simulink library "DSCdq_Library"  (R2018a)
settings: Solver=VariableStepAuto  StartTime=0.0  StopTime=10.0  RelTol=1e-3
values from neighbouring files (symbols this model uses):
  Fcutout = 1000    [Application_Script.m]
  Fmin = 40    [Application_Script.m]
  Fn = 60    [Application_Script.m]    (also in ShortPulse_Script.m)
  Fsw = 6000    [Application_Script.m]
  Kp = 4    [Application_Script.m]
  Ti = L/R    (= 0.0530516476973)    [Application_Script.m]
  Ts = Ts_control / 60    (= 9.25925925926e-07)    [Application_Script.m]    (also in ShortPulse_Script.m)
  Ts_control = 1/(300*Fn)    (= 5.55555555556e-05)    [Application_Script.m]    (also in ShortPulse_Script.m)
  X = 0.5    [Application_Script.m]
  zeta = 2^-0.5    (= 0.707106781187)    [Application_Script.m]    (also in ShortPulse_Script.m)
undefined symbols (not defined in the file or in its folder): DiscIntNeverNeededParam, ESS, fn, Iap, PCC, Sn, tctrl, Uanp
libraries: $bdroot x54, powerlib_meascontrol x33, powerlib x3, cstblocks x2, simulink x2, peTransforms x2
(part 1 of 2)
settings Model: Creator=daniemot  LastModifiedBy=daniemot

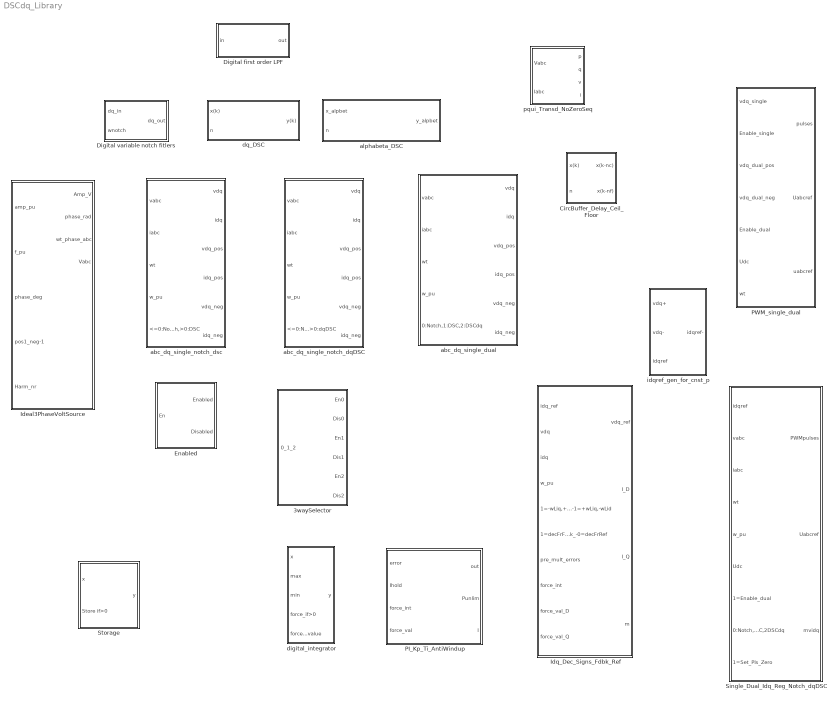
== system DSCdq_Library ==
  3waySelector : Subsystem  SystemSampleTime=Ts  mask(3 way selector){}
      mask Display: fprintf('Selector');
  CircBuffer_Delay_Ceil_Floor : Subsystem  TreatAsAtomicUnit=on  SystemSampleTime=Ts  mask(Circular buffer with two variable delays (ceiling and floor)){Ts=Ts, nmax=200}
      mask prompts: Ts "Sampling time [s]"; nmax "Circular buffer length"
      mask help:
      | Circular Buffer
      | By: Mota
      | Revision history:	2021-07-16: first release
      |
      | Interface
      | Inputs
      | 	x : must be a vector pf two values
      | 	n : delay in samples (float, ideal delay is time was continuous)
      | 	nmax : max size of circular buffer, ONLY used in FIRST CYCLE
      |
      | Output
      | 	yc = x(k - ceil(n))
      | 	yf = x(k - floor(n))
  Digital first order LPF : Subsystem  mask(Digital first-order low-pass filter){Ts=tctrl, fcutout=fn/2^0.5}
      mask prompts: Ts "Sample times [s]"; fcutout "Cutout frequency [Hz]"
      mask help:
      | Continuous time transfer function:  1/(1 + s T)
      | 	where T [s] = 1 / (2 pi fcutout [Hz]).
      |
      | Actual digital transfer function:   alpha / (1 + ( alpha -1) z^{-1} )
      | 	with eq. of diffs.: y = alpha x + (1 - alpha) y z^{-1}
      | 	where alpha = Ts / ( 1/(2 pi fcutout) + Ts)
      mask Display: fprintf('1/(1+sT)');
  Digital variable notch fitlers : Subsystem  mask{Ts=Ts, zeta=0.707}
      mask prompts: Ts "Sampling time [s]"; zeta "Damping factor zeta for notches"
  Enabled : Subsystem  SystemSampleTime=Ts  mask(Enabled block){}
      mask help:
      | if En > 0
      |     Enabled = 1;
      |     Disabled = 0;
      | else
      |     Enabled = 0;
      |     Disabled = 1;
      | end
      mask Display: fprintf('Enable');
  Ideal3PhaseVoltSource : Subsystem  mask(Three-phase ideal voltage source){BaseAmp=1, fn=50}
      mask prompts: BaseAmp "Base phase-to-neutral amplitude [V]"; fn "Base frequency [Hz]"
      mask help:
      | Three-phase balanced ideal voltage source with neutral point not connected.
      |
      | The voltage source can be connected in series with others.
      |
      | va [V] = amp_pu*BaseAmp*sin(2*pi*(f_pu/s)*Harm_nr + Harm_nr*phase_deg*pi/180)
      | vb [V] = ... + Harm_nr*Ph_b_sign*2*pi/3)
      | vc [V] = ... + Harm_nr*Ph_c_sign*2*pi/3)
      |
      | If Pos1_Neg-1 = 1
      | 	Ph_b_sign = -1
      | 	Ph_c_sign = +1
      |
      | If Pos1_Neg-1 = -1
      | 	Ph_b_sign = +1
      | 	Ph_c_sign = -1
  Idq_Dec_Signs_Fdbk_Ref : Subsystem  mask(Idq Controller - PI regulator with anti-windup){Ts=Ts_control, fn=50, Kp=0.4, Ti=0.13, L=0.3, PI_max=1.5, PI_min=-1.5, TrafoPhaseComp=0}
      mask prompts: Ts "Sampling time [s]"; fn "Rated frequency: fn [Hz]"; Kp "Proportional gain: Kp [pu]"; Ti "Integral time: Ti [s]"; L "DQ decoupl. inductance: L [pu]"; PI_max "Maximum output [pu]"; PI_min "Minimum output [pu]"; TrafoPhaseComp "Transformer phase compensation [rad]"
      mask help:
      | Idq Controller
      | Discrete PI regulator with forward Euler approximation for the integrator.
      | Transfer function: 	Kp (1 + sTi) / (sTi)
      | The anti-windup freezes the integrator if the unlimited output of the PI goes beyond the limits.
      |
      | Phase compensation for transformer winding: PhaseTrafoComp
  PI_Kp_Ti_AntiWindup : Subsystem  TreatAsAtomicUnit=on  SystemSampleTime=Ts  mask(PI regulator with anti-windup){Ts=0.001, Kp=10, Ti=1, PI_max=1, PI_min=-1}
      mask prompts: Ts "Sampling time [s]"; Kp "Proportional gain: Kp [pu]"; Ti "Integral time: Ti [s]"; PI_max "Maximum output [pu]"; PI_min "Minimum output [pu]"
      mask help:
      | Discrete PI regulator with forward Euler approximation for the integrator.
      |
      | Transfer function:
      | 	Kp (1 + sTi) / (sTi)
      |
      | The anti-windup freezes the integrator if the unlimited output of the PI goes beyond the limits.
      mask Display: fprintf('Kp(1+1/(sTi))');
  PWM_single_dual : Subsystem  mask(Scaling of vdq ref and PWM gate generation){fsw=50, Ts=1/200000, Uabp=1000, PWM_Ini_Phase=90}
      mask prompts: fsw "Switching frequency [Hz]"; Ts "Sampling time [s]"; Uabp "Rated peak line voltage [V]"; PWM_Ini_Phase "PWM carrier initial phase [degrees]"
      mask help:
      | Scales vdq_ref by: U_line_peak / Udc
      |
      | Add third harmonic to uabc_ref for overmodulation
  Single_Dual_Idq_Reg_Notch_dqDSC : Subsystem  mask(Notch based dual dq current regulator){Ts=Ts_control, fgrid=Fn, fmin=Fmin, zetanotch=zeta, fcutout=Fcutout, PI_Kp=Kp, PI_Ti=Ti, PI_X=X, PI_max=1.5, PI_min=-1.5, PWM_Ts=Ts, PWM_fsw=Fsw, PWM_Uabp=3^0.5, PWM_Ini=90}
      mask prompts: Ts "Sampling time controller [s]"; fgrid "Grid frequency [Hz]"; fmin "Min. acceptable grid freq. [Hz]"; zetanotch "Damping notch filters"; fcutout "Cutout freq. low pass for noise [Hz]"; PI_Kp "Proportional gain Kp [pu/pu]"; PI_Ti "Integrator time Ti [s]"; PI_X "Decoupling reactance X [pu]"; PI_max "PI max [pu]"; PI_min "PI min [pu]"; PWM_Ts "Sampling time PWM [s]"; PWM_fsw "Switching frequency [Hz]"; PWM_Uabp "Rated peak line voltage [V]"; PWM_Ini "Initial phase of carrier [degrees]"
      mask help: To be used with "abc -> dq" and "acb -> dq" transformations. When va = V sin (wt), vb = V sin (wt-120), vc = V sin (wt+120), -> vd = V vq=0.
      mask DialogControl Container2 Prompt: Transducers
      mask DialogControl Container7 Prompt: PI regulator
      mask DialogControl Container5 Prompt: PWM
  Storage : Subsystem  SystemSampleTime=Ts  mask(Storage block){}
      mask help:
      | if Store ==1
      |     Output = Input;
      | else
      |     Output = old ouptut;
      | end
      mask Display: fprintf('Store');
  abc_dq_single_dual : Subsystem  mask(abc->dq with Matlab){Ts=0.001, fn=50, fmin=40, zeta=0.707}
      mask prompts: Ts "Sampling time [s]"; fn "Grid frequency [Hz]"; fmin "Min. acceptable grid freq. [Hz]"; zeta "Zeta for notch filters"
      mask help:
      | To be done
      |
      | Max buffer size for DSC 500 samples
  abc_dq_single_notch_dqDSC : Subsystem  mask(abc->dq with Matlab){Ts=0.001, fn=50, fmin=40, zeta=0.707}
      mask prompts: Ts "Sampling time [s]"; fn "Grid frequency [Hz]"; fmin "Min. acceptable grid freq. [Hz]"; zeta "Zeta for notch filters"
      mask help:
      | To be done
      |
      | Max buffer size for DSC 500 samples
  abc_dq_single_notch_dsc : Subsystem  mask(abc->dq with Matlab){Ts=0.001, fn=50, fmin=40, zeta=0.707}
      mask prompts: Ts "Sampling time [s]"; fn "Rated grid frequency [Hz]"; fmin "Min. acceptable grid freq. [Hz]"; zeta "Zeta for notch filters"
      mask help:
      | To be done
      |
      | Max buffer size for DSC 500 samples
  alphabeta_DSC : Subsystem  mask{Ts=Ts, nmax=200}
      mask prompts: Ts "Sample times [s]"; nmax "Maximum delay nmax:"
      mask Display: fprintf('y(k)=0.5(x(k)+jx(k-n))');
  digital_integrator : Subsystem  SystemSampleTime=Ts  mask(Digital integrator){Ts=tctrl}
      mask prompts: Ts "Sample times [s]"
      mask help:
      | Forward Euler method: as in matlab help
      | 	y(n) = y(n-1) + Ts(n-1)*x(n-1)
      | uset it to avoid algebraic loops
      |
      | All inputs are stored in states, so there is no direct feedthrough. GAMBIARRA for avoiding algebraic loops, see https://www.mathworks.com/help/simulink/ug/integration-considerations-for-matlab-function-blocks.html
      |
      | Inputs
      |    x: input to the integrator
      |    max: max value for integrator
      |    min: min value for integrator
      |    force: if>=1 sets integrator to forceval
      |    forceval: see line above (max and min are respected
      |    Ts: sampling time
      | Output
      |    y: output of the integrator
      mask Display: fprintf('1/s');
  dq_DSC : Subsystem  mask{Ts=Ts, nmax=200}
      mask prompts: Ts "Sample times [s]"; nmax "Maximum delay nmax:"
      mask Display: fprintf('y(k)=0.5(x(k)+x(k-n))');
  idqref_gen_for_cnst_p : Subsystem  mask(idq reference gen for neg. seq. controller){Ts_control=Ts_control}
      mask prompts: Ts_control "Sampling time [s]"
      mask help:
      | Calculation of the negative sequence references for removing active power second harmonic oscillations.
      | Reactive power is allowed to oscillated with second harmonic.
      |
      | To be used with "abc -> dq" and "acb -> dq" transformations. When va = V sin (wt), vb = V sin (wt-120), vc = V sin (wt+120), -> vd = V vq=0.
      |
      | In "expanded" matrix form
      | | idn | = - | -vdp  +vqp |^{-1} * | -vdn  +vqn | * | idp |
      | | iqn | =   | +vqp  +vdp |        | -vdn  +vqn |   | idq |
      | In matrix form
      | idqn  = - vdqp^{-1} * vdqn * idqp
      |
      | Not tested for "abc (-omega) -> dq" (which I think is the formulation of Chaudhary 2012.
      | Derived independently from, but later noticed that it was proposed by Chaudhary in 2012 at "Negative Sequence Current Control in Wind Power Plants With VSC-HVDC Connection", check eq. (11).
  pqui_Transd_NoZeroSeq : Subsystem  mask(u i p q transducer - No zero sequence){Sn=Sn, Uanp=Uanp, Iap=Iap}
      mask prompts: Sn "Rated three-phase apparent power [VA]"; Uanp "Rated peak phase-to-groud voltage [V]"; Iap "Rated peak line current [A]"
      mask help:
      | Loosely based on Akagi 1984, but with Clarke Transformation for both the current and voltage
      | 	v  = (valpha^2 + vbeta^2)^0.5 / V_phase_peak
      | 	i   = (ialpha^2 + ibeta^2)^0.5 / I_line_peak
      | 	p  = 3/2 * (valpha ialpha +vbeta ibeta) / Sn
      | 	q  = 3/2 * (-valpha ibeta +vbeta ialpha) / Sn

== system DSCdq_Library/3waySelector ==
  0_1_2 : Inport
  MATLAB Function : MATLAB Function  SystemSampleTime=Ts
      settings: RTWSystemCode=Inline
  En0 : Outport
  Dis0 : Outport  Port=2
  En1 : Outport  Port=3
  Dis1 : Outport  Port=4
  En2 : Outport  Port=5
  Dis2 : Outport  Port=6
  wires:
  0_1_2/1 -> MATLAB Function/1(In)
  MATLAB Function/1(En0) -> En0/1
  MATLAB Function/2(Dis0) -> Dis0/1
  MATLAB Function/3(En1) -> En1/1
  MATLAB Function/4(Dis1) -> Dis1/1
  MATLAB Function/5(En2) -> En2/1
  MATLAB Function/6(Dis2) -> Dis2/1

== system DSCdq_Library/CircBuffer_Delay_Ceil_Floor ==
  x(k) : Inport
  n : Inport  Port=2
  Constant1 : Constant  Value=nmax
  MATLAB Function : MATLAB Function  TreatAsAtomicUnit=on  SystemSampleTime=Ts
  x(k-nc) : Outport
  x(k-nf) : Outport  Port=2
  wires:
  n/1 -> MATLAB Function/2(n)  "n"
  MATLAB Function/2(yf) -> x(k-nf)/1  "x(k-nf)"
  x(k)/1 -> MATLAB Function/1(x)  "x(k)"
  MATLAB Function/1(yc) -> x(k-nc)/1  "x(k-nc)"
  Constant1/1 -> MATLAB Function/3(nmax)

== system DSCdq_Library/Digital first order LPF ==
  note: Transfer function: alpha / ( 1 + ( alpha -1 ) z^{-1} )
  note: alpha = Ts / ( 1/(2 pi fcutout) + Ts )
  note: y = alpha x + ( 1 - alpha) y z^{-1}
  in : Inport
  Add7 : Sum  Commented=on  Inputs=+-
  Discrete Filter : DiscreteFilter  Numerator=[Ts/(1/(2*pi*fcutout)+Ts)]  Denominator=[1 Ts/(1/(2*pi*fcutout)+Ts)-1]  SampleTime=Ts
  Discrete-Time Integrator : DiscreteIntegrator  Commented=on  IntegratorMethod=Integration: Trapezoidal  SampleTime=Ts  ICPrevOutput=DiscIntNeverNeededParam  ICPrevScaledInput=DiscIntNeverNeededParam
  Gain6 : Gain  Commented=on  Gain=2*pi*fcutout
  Rate Transition3 : RateTransition  OutPortSampleTime=Ts
  out : Outport
  wires:
  Add7/1 -> Gain6/1
  Discrete-Time Integrator/1 -> Add7/2
  in/1 -> Rate Transition3/1
  Gain6/1 -> Discrete-Time Integrator/1
  Rate Transition3/1 -> Add7/1, Discrete Filter/1
  Discrete Filter/1 -> out/1

== system DSCdq_Library/Digital variable notch fitlers ==
  dq_in : Inport
  wnotch : Inport  Port=2
  Constant : Constant  Value=0
  Constant1 : Constant  Value=zeta
  Constant2 : Constant  Value=0
  Constant3 : Constant  Value=zeta
  Demux : Demux  Outputs=2
  Discrete Varying Notch : cstblocks/Linear Parameter Varying/Discrete Varying Notch  w0=0  Ts=Ts
      settings: SourceProductName=Control System Toolbox  SourceProductBaseCode=CT
  Discrete Varying Notch1 : cstblocks/Linear Parameter Varying/Discrete Varying Notch  w0=0  Ts=Ts
      settings: SourceProductName=Control System Toolbox  SourceProductBaseCode=CT
  Mux : Mux  Inputs=2
  dq_out : Outport
  wires:
  Constant/1 -> Discrete Varying Notch/3
  Constant1/1 -> Discrete Varying Notch/4
  Demux/2 -> Discrete Varying Notch1/1
  dq_in/1 -> Demux/1
  Constant2/1 -> Discrete Varying Notch1/3
  wnotch/1 -> Discrete Varying Notch1/2, Discrete Varying Notch/2
  Constant3/1 -> Discrete Varying Notch1/4
  Demux/1 -> Discrete Varying Notch/1
  Discrete Varying Notch/1 -> Mux/1
  Mux/1 -> dq_out/1
  Discrete Varying Notch1/1 -> Mux/2

== system DSCdq_Library/Enabled ==
  En : Inport
  MATLAB Function : MATLAB Function  SystemSampleTime=Ts
      settings: RTWSystemCode=Inline
  Enabled : Outport
  Disabled : Outport  Port=2
  wires:
  En/1 -> MATLAB Function/1(En)
  MATLAB Function/1(Enabled) -> Enabled/1
  MATLAB Function/2(Disabled) -> Disabled/1

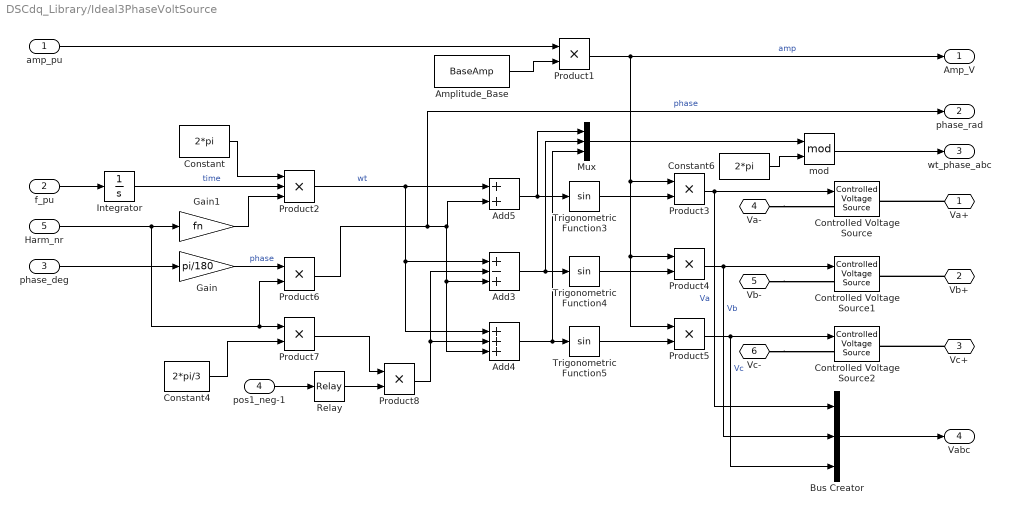
== system DSCdq_Library/Ideal3PhaseVoltSource ==
  amp_pu : Inport
  f_pu : Inport  Port=2
  phase_deg : Inport  Port=3
  pos1_neg-1 : Inport  Port=4
  Harm_nr : Inport  Port=5
  Add3 : Sum  Inputs=+-+
  Add4 : Sum  Inputs=+++
  Add5 : Sum
  Amplitude_Base : Constant  Value=BaseAmp
  Bus Creator : BusCreator  Inputs=3
  Constant : Constant  Value=2*pi
  Constant4 : Constant  Value=2*pi/3
  Constant6 : Constant  Value=2*pi
  Controlled Voltage Source : powerlib/Electrical Sources/Controlled Voltage Source  Initialize=off  Source_Type=AC  Amplitude=ESS.LSC.Ub*(2/3)^0.5  Phase=0  Frequency=PCC.fn  Measurements=None
  Controlled Voltage Source1 : powerlib/Electrical Sources/Controlled Voltage Source  Initialize=off  Source_Type=AC  Amplitude=ESS.LSC.Ub*(2/3)^0.5  Phase=-120  Frequency=PCC.fn  Measurements=None
  Controlled Voltage Source2 : powerlib/Electrical Sources/Controlled Voltage Source  Initialize=off  Source_Type=AC  Amplitude=ESS.LSC.Ub*(2/3)^0.5  Phase=120  Frequency=PCC.fn  Measurements=None
  Gain : Gain  Gain=pi/180
  Gain1 : Gain  Gain=fn
  Integrator : Integrator
  Mux : Mux  Inputs=3
  Product{1,3..8} (7 alike) : Product
  Product2 : Product  Inputs=3
  Relay : Relay  OnSwitchValue=0  OffSwitchValue=-0.1  OffOutputValue=-1
  Trigonometric Function3 : Trigonometry
  Trigonometric Function4 : Trigonometry
  Trigonometric Function5 : Trigonometry
  mod : Math  Operator=mod  SaturateOnIntegerOverflow=on
  Va+ : PMIOPort  Side=Right
  Vb+ : PMIOPort  Port=2  Side=Right
  Vc+ : PMIOPort  Port=3  Side=Right
  Va- : PMIOPort  Port=4  Side=Right
  Vb- : PMIOPort  Port=5  Side=Right
  Vc- : PMIOPort  Port=6  Side=Right
  Amp_V : Outport
  phase_rad : Outport  Port=2
  wt_phase_abc : Outport  Port=3
  Vabc : Outport  Port=4
  wires:
  Add4/1 -> Mux/3, Trigonometric Function5/1
  Product6/1 -> phase_rad/1, Add4/3, Add3/3, Add5/2  "phase"
  Add3/1 -> Mux/2, Trigonometric Function4/1
  pos1_neg-1/1 -> Relay/1
  Product3/1 -> Bus Creator/1, Controlled Voltage Source/1  "Va"
  amp_pu/1 -> Product1/1
  Product8/1 -> Add3/2, Add4/2
  Product5/1 -> Bus Creator/3, Controlled Voltage Source2/1  "Vc"
  Product4/1 -> Bus Creator/2, Controlled Voltage Source1/1  "Vb"
  Amplitude_Base/1 -> Product1/2
  Product7/1 -> Product8/1
  Product1/1 -> Product5/1, Product4/1, Product3/1, Amp_V/1  "amp"
  Relay/1 -> Product8/2
  Trigonometric Function3/1 -> Product3/2
  Product2/1 -> Add5/1, Add4/1, Add3/1  "wt"
  Trigonometric Function5/1 -> Product5/2
  Add5/1 -> Mux/1, Trigonometric Function3/1
  Trigonometric Function4/1 -> Product4/2
  phase_deg/1 -> Gain/1
  f_pu/1 -> Integrator/1
  Constant/1 -> Product2/1
  Gain1/1 -> Product2/3
  Bus Creator/1 -> Vabc/1
  Constant6/1 -> mod/2
  mod/1 -> wt_phase_abc/1
  Gain/1 -> Product6/1  "phase"
  Constant4/1 -> Product7/2
  Mux/1 -> mod/1
  Harm_nr/1 -> Product7/1, Product6/2, Gain1/1
  Integrator/1 -> Product2/2  "time"
  connections:
  Vb+/RConn1 -- Controlled Voltage Source1/RConn1
  Vc+/RConn1 -- Controlled Voltage Source2/RConn1
  Va+/RConn1 -- Controlled Voltage Source/RConn1
  Va-/RConn1 -- Controlled Voltage Source/LConn1
  Vb-/RConn1 -- Controlled Voltage Source1/LConn1
  Vc-/RConn1 -- Controlled Voltage Source2/LConn1

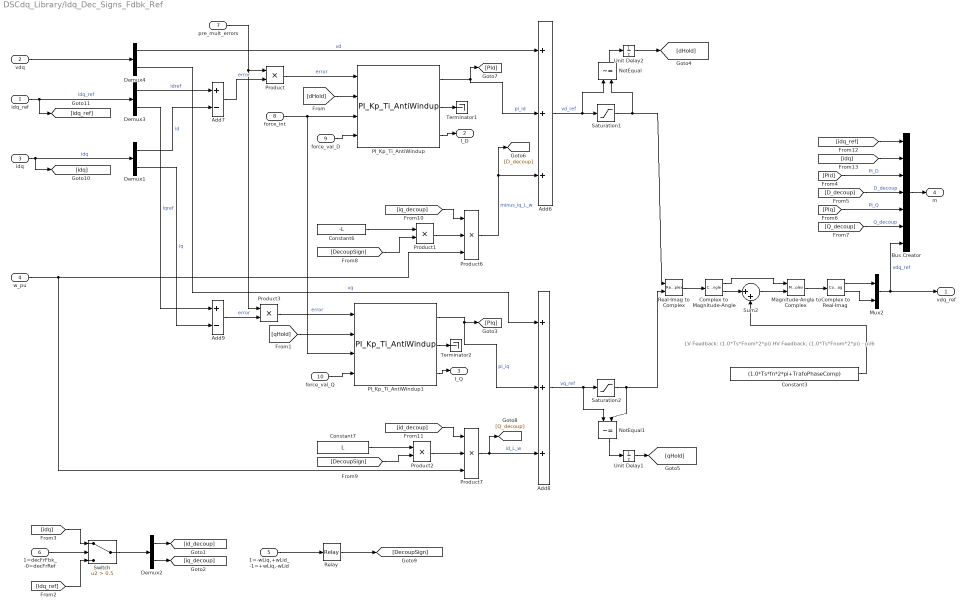
== system DSCdq_Library/Idq_Dec_Signs_Fdbk_Ref ==
  note: LV Feedback: (1.0*Ts*Fnom*2*pi)
      | HV Feedback: (1.0*Ts*Fnom*2*pi) - pi/6
  idq_ref : Inport
  vdq : Inport  Port=2
  idq : Inport  Port=3
  w_pu : Inport  Port=4
  1=-wLiq,+wLid_-1=+wLiq,-wLid : Inport  Port=5
  1=decFrFbk_-0=decFrRef : Inport  Port=6
  pre_mult_errors : Inport  Port=7
  force_int : Inport  Port=8
  force_val_D : Inport  Port=9
  force_val_Q : Inport  Port=10
  Add6 : Sum  Inputs=+++
  Add7 : Sum  Inputs=+-
  Add8 : Sum  Inputs=+++
  Add9 : Sum  Inputs=+-
  Bus Creator : BusCreator  Inputs=7
  Complex to Magnitude-Angle : ComplexToMagnitudeAngle
  Complex to Real-Imag : ComplexToRealImag
  Constant3 : Constant  Value=(1.0*Ts*fn*2*pi+TrafoPhaseComp)  SampleTime=Ts
  Constant6 : Constant  Value=-L  SampleTime=Ts
  Constant7 : Constant  Value=L  SampleTime=Ts
  Demux{1..4} (4 alike) : Demux  Outputs=2
  Magnitude-Angle to Complex : MagnitudeAngleToComplex
  Mux2 : Mux  Inputs=2
  NotEqual : RelationalOperator  Operator=~=  OutDataTypeStr=boolean  RndMeth=Simplest
  NotEqual1 : RelationalOperator  Operator=~=  OutDataTypeStr=boolean  RndMeth=Simplest
  PI_Kp_Ti_AntiWindup : $bdroot/PI_Kp_Ti_AntiWindup  Ts=Ts  Kp=Kp  Ti=Ti  PI_max=PI_max  PI_min=PI_min
  PI_Kp_Ti_AntiWindup1 : $bdroot/PI_Kp_Ti_AntiWindup  Ts=Ts  Kp=Kp  Ti=Ti  PI_max=PI_max  PI_min=PI_min
  Product : Product
  Product1 : Product  RndMeth=Zero
  Product2 : Product  RndMeth=Zero
  Product3 : Product
  Product6 : Product  Inputs=3  RndMeth=Zero
  Product7 : Product  Inputs=3  RndMeth=Zero
  Real-Imag to Complex : RealImagToComplex
  Relay : Relay  OnSwitchValue=0  OffSwitchValue=-0.1  OffOutputValue=-1
  Saturation1 : Saturate  UpperLimit=PI_max  LowerLimit=PI_min
  Saturation2 : Saturate  UpperLimit=PI_max  LowerLimit=PI_min
  Sum2 : Sum  Inputs=|++
  Switch : Switch  Criteria=u2 > Threshold  Threshold=0.5
  Terminator1 : Terminator
  Terminator2 : Terminator
  Unit Delay1 : UnitDelay  SampleTime=Ts
  Unit Delay2 : UnitDelay  SampleTime=Ts
  vdq_ref : Outport
  I_D : Outport  Port=2
  I_Q : Outport  Port=3
  m : Outport  Port=4
  wires:
  PI_Kp_Ti_AntiWindup1/1 -> Add8/2, [PIq]  "pi_iq"
  PI_Kp_Ti_AntiWindup1/2 -> Terminator2/1
  PI_Kp_Ti_AntiWindup/2 -> Terminator1/1
  w_pu/1 -> Product7/3, Product6/3
  Product3/1 -> PI_Kp_Ti_AntiWindup1/1  "error"
  PI_Kp_Ti_AntiWindup/1 -> [PId], Add6/2  "pi_id"
  Constant6/1 -> Product1/1
  Constant7/1 -> Product2/1
  Demux1/1 -> Add7/2  "id"
  Product7/1 -> [Q_decoup], Add8/3  "id_L_w"
  Demux4/1 -> Add6/1  "vd"
  Product/1 -> PI_Kp_Ti_AntiWindup/1  "error"
  Demux1/2 -> Add9/2  "iq"
  Product6/1 -> [D_decoup], Add6/3  "minus_iq_L_w"
  PI_Kp_Ti_AntiWindup1/3 -> I_Q/1
  PI_Kp_Ti_AntiWindup/3 -> I_D/1
  Demux4/2 -> Add8/1  "vq"
  Mux2/1 -> Bus Creator/7, vdq_ref/1  "vdq_ref"
  idq/1 -> [idq], Demux1/1  "idq"
  vdq/1 -> Demux4/1
  Add8/1 -> NotEqual1/1, Saturation2/1  "vq_ref"
  Add6/1 -> NotEqual/1, Saturation1/1  "vd_ref"
  idq_ref/1 -> [idq_ref], Demux3/1  "idq_ref"
  Demux3/1 -> Add7/1  "idref"
  Demux3/2 -> Add9/1  "iqref"
  Magnitude-Angle to Complex/1 -> Complex to Real-Imag/1
  Real-Imag to Complex/1 -> Complex to Magnitude-Angle/1
  Complex to Magnitude-Angle/1 -> Magnitude-Angle to Complex/1
  Complex to Magnitude-Angle/2 -> Sum2/1
  Sum2/1 -> Magnitude-Angle to Complex/2
  Constant3/1 -> Sum2/2
  Complex to Real-Imag/1 -> Mux2/1
  Complex to Real-Imag/2 -> Mux2/2
  [PId] -> Bus Creator/3  "PI_D"
  [D_decoup] -> Bus Creator/4  "D_decoup"
  [PIq] -> Bus Creator/5  "PI_Q"
  Bus Creator/1 -> m/1
  [Q_decoup] -> Bus Creator/6  "Q_decoup"
  Saturation1/1 -> NotEqual/2, Real-Imag to Complex/1
  NotEqual/1 -> Unit Delay2/1
  Saturation2/1 -> NotEqual1/2, Real-Imag to Complex/2
  NotEqual1/1 -> Unit Delay1/1
  Unit Delay2/1 -> [dHold]
  Unit Delay1/1 -> [qHold]
  [dHold] -> PI_Kp_Ti_AntiWindup/2
  [qHold] -> PI_Kp_Ti_AntiWindup1/2
  Relay/1 -> [DecoupSign]
  1=-wLiq,+wLid_-1=+wLiq,-wLid/1 -> Relay/1
  [DecoupSign] -> Product1/2
  Product1/1 -> Product6/2
  Product2/1 -> Product7/2
  [DecoupSign] -> Product2/2
  [idq_ref] -> Switch/3
  Demux2/2 -> [iq_decoup]
  1=decFrFbk_-0=decFrRef/1 -> Switch/2
  Demux2/1 -> [id_decoup]
  Switch/1 -> Demux2/1
  [idq] -> Switch/1
  [iq_decoup] -> Product6/1
  [id_decoup] -> Product7/1
  [idq_ref] -> Bus Creator/1
  [idq] -> Bus Creator/2
  force_int/1 -> PI_Kp_Ti_AntiWindup1/3, PI_Kp_Ti_AntiWindup/3
  force_val_D/1 -> PI_Kp_Ti_AntiWindup/4
  force_val_Q/1 -> PI_Kp_Ti_AntiWindup1/4
  Add9/1 -> Product3/2  "error"
  Add7/1 -> Product/2  "error"
  pre_mult_errors/1 -> Product3/1, Product/1

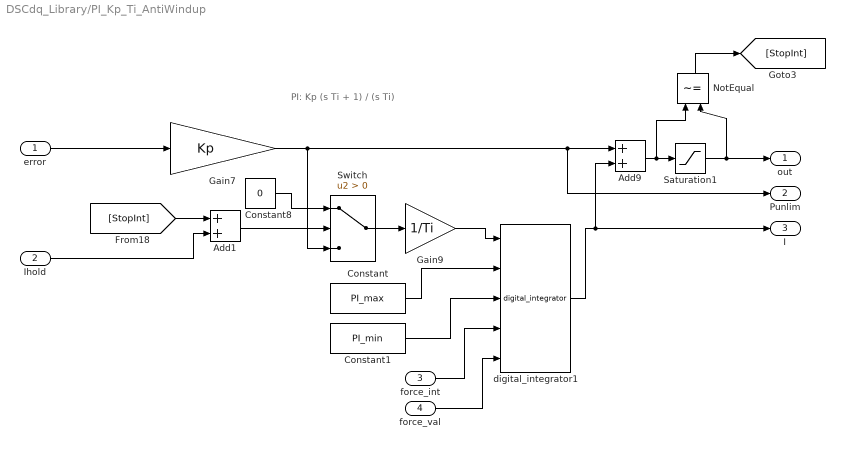
== system DSCdq_Library/PI_Kp_Ti_AntiWindup ==
  note: PI: Kp (s Ti + 1) / (s Ti)
  error : Inport
  Ihold : Inport  Port=2
  force_int : Inport  Port=3
  force_val : Inport  Port=4
  Add1 : Sum
  Add9 : Sum
  Constant : Constant  Value=PI_max
  Constant1 : Constant  Value=PI_min
  Constant8 : Constant  Value=0
  Gain7 : Gain  Gain=Kp
  Gain9 : Gain  Gain=1/Ti
  NotEqual : RelationalOperator  Operator=~=  OutDataTypeStr=boolean  RndMeth=Simplest
  Saturation1 : Saturate  UpperLimit=PI_max  LowerLimit=PI_min
  Switch : Switch  Criteria=u2 > Threshold
  digital_integrator1 : $bdroot/digital_integrator  Ts=Ts
  out : Outport
  Punlim : Outport  Port=2
  I : Outport  Port=3
  wires:
  NotEqual/1 -> [StopInt]
  Saturation1/1 -> out/1, NotEqual/2
  error/1 -> Gain7/1
  digital_integrator1/1 -> I/1, Add9/2
  Add1/1 -> Switch/2
  Constant8/1 -> Switch/1
  Gain7/1 -> Switch/3, Punlim/1, Add9/1
  Switch/1 -> Gain9/1
  Add9/1 -> NotEqual/1, Saturation1/1
  Gain9/1 -> digital_integrator1/1
  [StopInt] -> Add1/1
  Ihold/1 -> Add1/2
  Constant1/1 -> digital_integrator1/3
  force_int/1 -> digital_integrator1/4
  force_val/1 -> digital_integrator1/5
  Constant/1 -> digital_integrator1/2

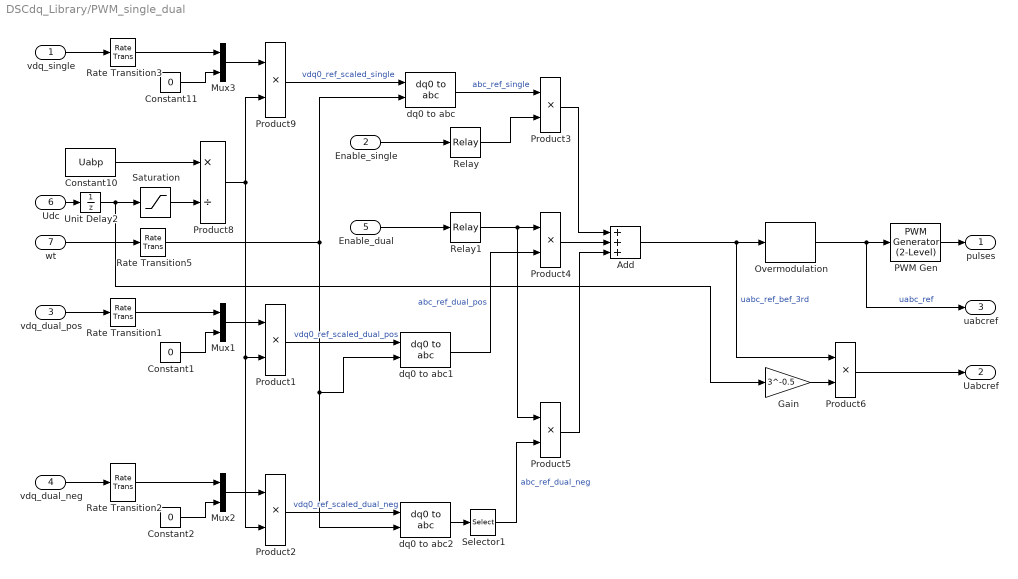
== system DSCdq_Library/PWM_single_dual ==
  vdq_single : Inport
  Enable_single : Inport  Port=2
  vdq_dual_pos : Inport  Port=3
  vdq_dual_neg : Inport  Port=4
  Enable_dual : Inport  Port=5
  Udc : Inport  Port=6
  wt : Inport  Port=7
  Add : Sum  Inputs=+++
  Constant1 : Constant  Value=0
  Constant10 : Constant  Value=Uabp
  Constant11 : Constant  Value=0
  Constant2 : Constant  Value=0
  Gain : Gain  Gain=3^-0.5
  Mux1 : Mux  Inputs=[2 1]
  Mux2 : Mux  Inputs=[2 1]
  Mux3 : Mux  Inputs=[2 1]
  Overmodulation : powerlib_meascontrol/Pulse & Signal Generators/Overmodulation  OverModType=Third harmonic
      settings: SourceProductName=Simscape Power Systems  SourceProductBaseCode=PS
  PWM Gen : powerlib_meascontrol/Pulse & Signal Generators/PWM Generator (2-Level)  ModulatorType=Three-phase bridge (6 pulses)  ModulatorMode=Unsynchronized  Fc=fsw  Pc=PWM_Ini_Phase  nF=27  MinMax="[ -1  1 ]"  SamplingTechnique=Asymmetrical regular (double edge)  ModulatingSignals=off  m=0.8  Freq=60  Phase=0  Ts=Ts  ShowCarrierOutport=off
      settings: SourceProductName=Simscape Power Systems
  Product{1..6,9} (7 alike) : Product  Inputs=**
  Product8 : Product  Inputs=*/
  Rate Transition{1..3,5} (4 alike) : RateTransition  OutPortSampleTime=Ts
  Relay : Relay  OnSwitchValue=0.6  OffSwitchValue=0.4
  Relay1 : Relay  OnSwitchValue=0.6  OffSwitchValue=0.4
  Saturation : Saturate  UpperLimit=10*Uabp  LowerLimit=0.001*Uabp
  Selector1 : Selector  InputPortWidth=3  IndexOptions=Index vector (dialog)  Indices=[1 3 2]  OutputSizes=1
  Unit Delay2 : UnitDelay  InitialCondition=Uabp  SampleTime=Ts
  dq0 to abc : powerlib_meascontrol/Transformations/dq0 to abc  Alignment=90 degrees behind phase A axis
  dq0 to abc1 : powerlib_meascontrol/Transformations/dq0 to abc  Alignment=90 degrees behind phase A axis
  dq0 to abc2 : powerlib_meascontrol/Transformations/dq0 to abc  Alignment=90 degrees behind phase A axis
  pulses : Outport
  Uabcref : Outport  Port=2
  uabcref : Outport  Port=3
  wires:
  dq0 to abc1/1 -> Product4/2  "abc_ref_dual_pos"
  Rate Transition5/1 -> dq0 to abc/2, dq0 to abc1/2, dq0 to abc2/2
  Product1/1 -> dq0 to abc1/1  "vdq0_ref_scaled_dual_pos"
  vdq_dual_pos/1 -> Rate Transition1/1
  Constant1/1 -> Mux1/2
  Mux1/1 -> Product1/1
  Rate Transition1/1 -> Mux1/1
  Product6/1 -> Uabcref/1
  vdq_single/1 -> Rate Transition3/1
  PWM Gen/1 -> pulses/1
  Udc/1 -> Unit Delay2/1
  Overmodulation/1 -> uabcref/1, PWM Gen/1  "uabc_ref"
  Constant10/1 -> Product8/1
  wt/1 -> Rate Transition5/1
  Rate Transition3/1 -> Mux3/1
  Mux3/1 -> Product9/1
  Unit Delay2/1 -> Gain/1, Saturation/1
  Product9/1 -> dq0 to abc/1  "vdq0_ref_scaled_single"
  Constant11/1 -> Mux3/2
  dq0 to abc/1 -> Product3/1  "abc_ref_single"
  Enable_single/1 -> Relay/1
  Enable_dual/1 -> Relay1/1
  Add/1 -> Product6/1, Overmodulation/1  "uabc_ref_bef_3rd"
  Saturation/1 -> Product8/2
  Product8/1 -> Product2/2, Product1/2, Product9/2
  Rate Transition2/1 -> Mux2/1
  vdq_dual_neg/1 -> Rate Transition2/1
  Mux2/1 -> Product2/1
  Constant2/1 -> Mux2/2
  Product2/1 -> dq0 to abc2/1  "vdq0_ref_scaled_dual_neg"
  dq0 to abc2/1 -> Selector1/1
  Selector1/1 -> Product5/2  "abc_ref_dual_neg"
  Relay/1 -> Product3/2
  Product3/1 -> Add/1
  Product4/1 -> Add/2
  Relay1/1 -> Product5/1, Product4/1
  Product5/1 -> Add/3
  Gain/1 -> Product6/2

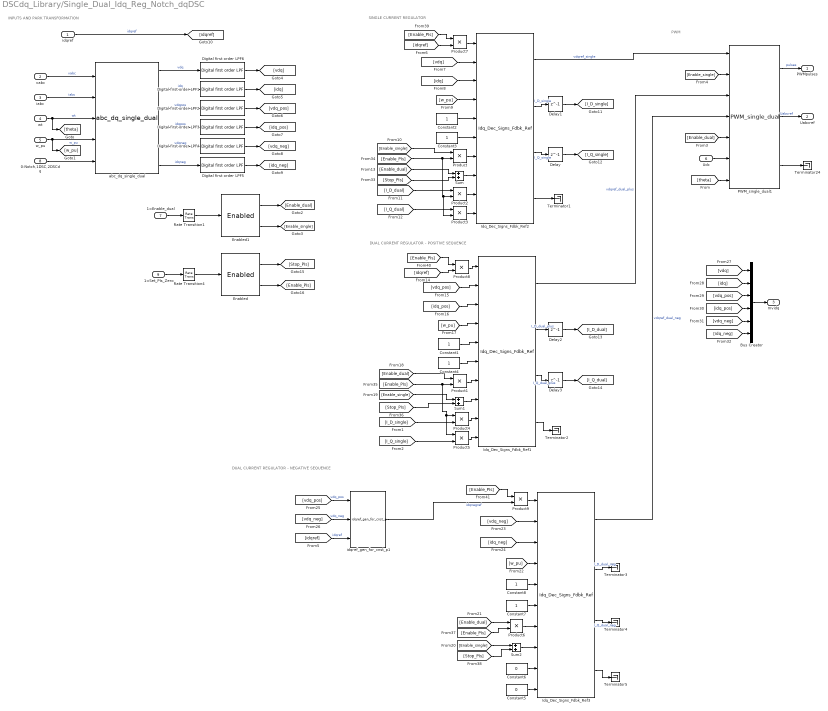
== system DSCdq_Library/Single_Dual_Idq_Reg_Notch_dqDSC ==
  note: PWM
  note: DUAL CURRENT REGULATOR - NEGATIVE SEQUENCE
  note: DUAL CURRENT REGULATOR - POSITIVE SEQUENCE
  note: SINGLE CURRENT REGULATOR
  note: INPUTS AND PARK TRANSFORMATION
  idqref : Inport
  vabc : Inport  Port=2
  iabc : Inport  Port=3
  wt : Inport  Port=4
  w_pu : Inport  Port=5
  Udc : Inport  Port=6
  1=Enable_dual : Inport  Port=7
  0:Notch,1DSC,2DSCdq : Inport  Port=8
  1=Set_PIs_Zero : Inport  Port=9
  Bus Creator : BusCreator  Inputs=6
  Constant{1..4,7..8} (6 alike) : Constant
  Constant5 : Constant  Value=0
  Constant6 : Constant  Value=0
  Delay{,1..3} (4 alike) : Delay  DelayLength=1  InitialCondition=0  SampleTime=Ts
  Digital first order LPF{1..6} (6 alike) : $bdroot/Digital first order LPF  Ts=Ts  fcutout=fcutout
  Enabled : $bdroot/Enabled
  Enabled1 : $bdroot/Enabled
  Idq_Dec_Signs_Fdbk_Ref1 : $bdroot/Idq_Dec_Signs_Fdbk_Ref  Ts=Ts  fn=fgrid  Kp=PI_Kp  Ti=PI_Ti  L=PI_X  PI_max=PI_max  PI_min=PI_min  TrafoPhaseComp=0
  Idq_Dec_Signs_Fdbk_Ref2 : $bdroot/Idq_Dec_Signs_Fdbk_Ref  Ts=Ts  fn=fgrid  Kp=PI_Kp  Ti=PI_Ti  L=PI_X  PI_max=PI_max  PI_min=PI_min  TrafoPhaseComp=0
  Idq_Dec_Signs_Fdbk_Ref3 : $bdroot/Idq_Dec_Signs_Fdbk_Ref  Ts=Ts  fn=fgrid  Kp=PI_Kp  Ti=PI_Ti  L=PI_X  PI_max=PI_max  PI_min=PI_min  TrafoPhaseComp=0
  PWM_single_dual1 : $bdroot/PWM_single_dual  fsw=PWM_fsw  Ts=PWM_Ts  Uabp=PWM_Uabp  PWM_Ini_Phase=PWM_Ini
  Product{,1..9} (10 alike) : Product
  Rate Transition1 : RateTransition  OutPortSampleTime=Ts
  Rate Transition4 : RateTransition  InitialCondition=1  OutPortSampleTime=Ts
  Sum : Sum
  Sum1 : Sum
  Sum2 : Sum
  Terminator{1..5,24} (6 alike) : Terminator
  abc_dq_single_dual : $bdroot/abc_dq_single_dual  Ts=Ts  fn=fgrid  fmin=fmin  zeta=zetanotch
  idqref_gen_for_cnst_p1 : $bdroot/idqref_gen_for_cnst_p  Ts_control=Ts
  PWMpulses : Outport
  Uabcref : Outport  Port=2
  mvidq : Outport  Port=3
  wires:
  [Enable_PIs] -> Product9/1
  Udc/1 -> PWM_single_dual1/6
  PWM_single_dual1/3 -> Terminator24/1
  PWM_single_dual1/2 -> Uabcref/1  "Uabcref"
  [idqref] -> idqref_gen_for_cnst_p1/3  "idqref"
  [theta] -> PWM_single_dual1/7
  PWM_single_dual1/1 -> PWMpulses/1  "pulses"
  [Enable_dual] -> PWM_single_dual1/5
  [Enable_single] -> PWM_single_dual1/2
  vabc/1 -> abc_dq_single_dual/1  "vabc"
  iabc/1 -> abc_dq_single_dual/2  "iabc"
  wt/1 -> abc_dq_single_dual/3, [theta]  "wt"
  w_pu/1 -> abc_dq_single_dual/4, [w_pu]  "w_pu"
  abc_dq_single_dual/1 -> Digital first order LPF6/1  "vdq"
  abc_dq_single_dual/2 -> Digital first order LPF1/1  "idq"
  abc_dq_single_dual/3 -> Digital first order LPF2/1  "vdqpos"
  abc_dq_single_dual/4 -> Digital first order LPF3/1  "idqpos"
  abc_dq_single_dual/5 -> Digital first order LPF4/1  "vdqneg"
  abc_dq_single_dual/6 -> Digital first order LPF5/1  "idqneg"
  idqref/1 -> [idqref]  "idqref"
  [idqref] -> Product7/2
  [vdq] -> Idq_Dec_Signs_Fdbk_Ref2/2
  [idq] -> Idq_Dec_Signs_Fdbk_Ref2/3
  [w_pu] -> Idq_Dec_Signs_Fdbk_Ref2/4
  Constant2/1 -> Idq_Dec_Signs_Fdbk_Ref2/5
  Constant3/1 -> Idq_Dec_Signs_Fdbk_Ref2/6
  0:Notch,1DSC,2DSCdq/1 -> abc_dq_single_dual/5
  [Enable_single] -> Product/1
  Idq_Dec_Signs_Fdbk_Ref2/3 -> Delay/1  "I_Q_single"
  Idq_Dec_Signs_Fdbk_Ref2/2 -> Delay1/1  "I_D_single"
  Idq_Dec_Signs_Fdbk_Ref1/2 -> Delay2/1  "I_D_dual_plus"
  Idq_Dec_Signs_Fdbk_Ref1/3 -> Delay3/1  "I_Q_dual_plus"
  Delay1/1 -> [I_D_single]
  Delay/1 -> [I_Q_single]
  Delay2/1 -> [I_D_dual]
  Delay3/1 -> [I_Q_dual]
  [I_D_single] -> Product4/2
  [I_Q_single] -> Product5/2
  [I_D_dual] -> Product2/1
  [I_Q_dual] -> Product3/1
  [Enable_dual] -> Sum/1
  [idqref] -> Product8/2
  [vdq_pos] -> Idq_Dec_Signs_Fdbk_Ref1/2
  [idq_pos] -> Idq_Dec_Signs_Fdbk_Ref1/3
  [w_pu] -> Idq_Dec_Signs_Fdbk_Ref1/4
  Constant1/1 -> Idq_Dec_Signs_Fdbk_Ref1/5
  Constant4/1 -> Idq_Dec_Signs_Fdbk_Ref1/6
  [Enable_dual] -> Product1/1
  [Enable_single] -> Sum1/1
  Idq_Dec_Signs_Fdbk_Ref2/4 -> Terminator1/1
  Idq_Dec_Signs_Fdbk_Ref1/4 -> Terminator2/1
  Idq_Dec_Signs_Fdbk_Ref3/2 -> Terminator3/1  "I_D_dual_neg"
  Idq_Dec_Signs_Fdbk_Ref3/3 -> Terminator4/1  "I_Q_dual_neg"
  Idq_Dec_Signs_Fdbk_Ref3/4 -> Terminator5/1
  Constant5/1 -> Idq_Dec_Signs_Fdbk_Ref3/10
  Constant6/1 -> Idq_Dec_Signs_Fdbk_Ref3/9
  [Enable_single] -> Sum2/1
  [Enable_dual] -> Product6/1
  Constant7/1 -> Idq_Dec_Signs_Fdbk_Ref3/6
  Constant8/1 -> Idq_Dec_Signs_Fdbk_Ref3/5
  [w_pu] -> Idq_Dec_Signs_Fdbk_Ref3/4
  [vdq_neg] -> Idq_Dec_Signs_Fdbk_Ref3/2
  [idq_neg] -> Idq_Dec_Signs_Fdbk_Ref3/3
  [vdq_neg] -> idqref_gen_for_cnst_p1/2  "vdq_neg"
  idqref_gen_for_cnst_p1/1 -> Product9/2  "idqnegref"
  Idq_Dec_Signs_Fdbk_Ref2/1 -> PWM_single_dual1/1  "vdqref_single"
  Idq_Dec_Signs_Fdbk_Ref1/1 -> PWM_single_dual1/3  "vdqref_dual_plus"
  Idq_Dec_Signs_Fdbk_Ref3/1 -> PWM_single_dual1/4  "vdqref_dual_neg"
  Bus Creator/1 -> mvidq/1
  [vdq] -> Bus Creator/1
  [idq] -> Bus Creator/2
  [vdq_pos] -> Bus Creator/3
  [idq_pos] -> Bus Creator/4
  [vdq_neg] -> Bus Creator/5
  [idq_neg] -> Bus Creator/6
  1=Set_PIs_Zero/1 -> Rate Transition4/1
  Enabled/1 -> [Stop_PIs]
  Enabled/2 -> [Enable_PIs]
  [Enable_PIs] -> Product3/2, Product2/2, Product/2
  Product/1 -> Idq_Dec_Signs_Fdbk_Ref2/7
  Sum/1 -> Idq_Dec_Signs_Fdbk_Ref2/8
  Product3/1 -> Idq_Dec_Signs_Fdbk_Ref2/10
  [Stop_PIs] -> Sum/2
  Product2/1 -> Idq_Dec_Signs_Fdbk_Ref2/9
  Product1/1 -> Idq_Dec_Signs_Fdbk_Ref1/7
  [Enable_PIs] -> Product5/1, Product4/1, Product1/2
  Sum1/1 -> Idq_Dec_Signs_Fdbk_Ref1/8
  [Stop_PIs] -> Sum1/2
  Product5/1 -> Idq_Dec_Signs_Fdbk_Ref1/10
  Product4/1 -> Idq_Dec_Signs_Fdbk_Ref1/9
  [Enable_PIs] -> Product6/2
  Product6/1 -> Idq_Dec_Signs_Fdbk_Ref3/7
  [Stop_PIs] -> Sum2/2
  Sum2/1 -> Idq_Dec_Signs_Fdbk_Ref3/8
  [Enable_PIs] -> Product7/1
  Product7/1 -> Idq_Dec_Signs_Fdbk_Ref2/1
  [Enable_PIs] -> Product8/1
  Product8/1 -> Idq_Dec_Signs_Fdbk_Ref1/1
  Product9/1 -> Idq_Dec_Signs_Fdbk_Ref3/1
  Rate Transition4/1 -> Enabled/1
  Enabled1/1 -> [Enable_dual]
  Enabled1/2 -> [Enable_single]
  Rate Transition1/1 -> Enabled1/1
  1=Enable_dual/1 -> Rate Transition1/1
  [vdq_pos] -> idqref_gen_for_cnst_p1/1  "vdq_pos"
  Digital first order LPF6/1 -> [vdq]
  Digital first order LPF1/1 -> [idq]
  Digital first order LPF2/1 -> [vdq_pos]
  Digital first order LPF3/1 -> [idq_pos]
  Digital first order LPF4/1 -> [vdq_neg]
  Digital first order LPF5/1 -> [idq_neg]

== system DSCdq_Library/Storage ==
  x : Inport
  Store if>0 : Inport  Port=2
  MATLAB Function : MATLAB Function  SystemSampleTime=Ts
      settings: RTWSystemCode=Inline
  y : Outport
  wires:
  MATLAB Function/1(y) -> y/1
  x/1 -> MATLAB Function/1(x)
  Store if>0/1 -> MATLAB Function/2(store)

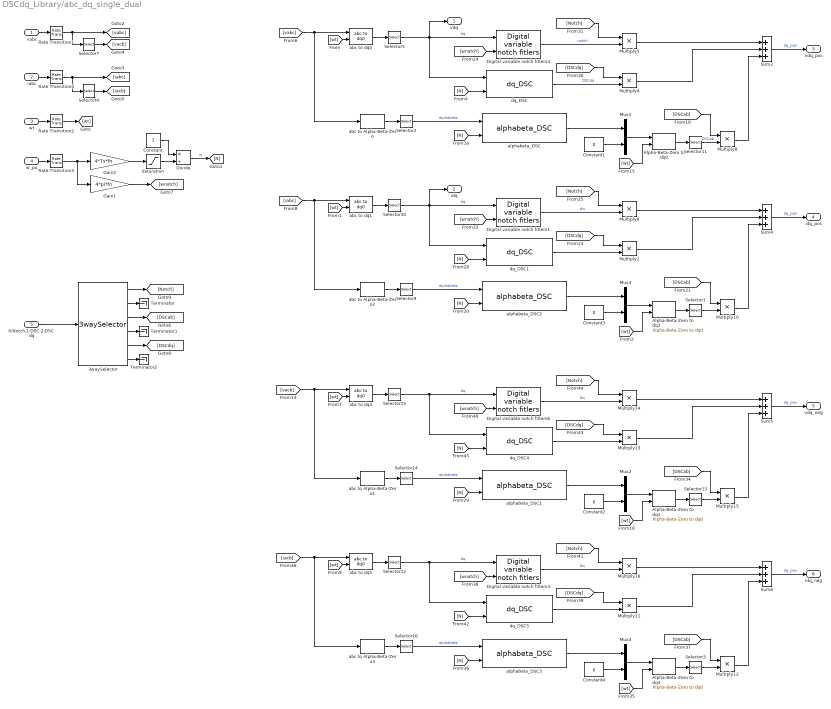
== system DSCdq_Library/abc_dq_single_dual ==
  vabc : Inport
  iabc : Inport  Port=2
  wt : Inport  Port=3
  w_pu : Inport  Port=4
  0:Notch,1:DSC,2:DSCdq : Inport  Port=5
  3waySelector : $bdroot/3waySelector
  Alpha-Beta-Zero to dq{0..3} (4 alike) : powerlib_meascontrol/Transformations/Alpha-Beta-Zero to dq0  Alignment=90 degrees behind phase A axis
      settings: SourceProductName=Simscape Power Systems
  Constant : Constant
  Constant{1..4} (4 alike) : Constant  Value=0
  Digital variable notch fitlers{1,3..4,6} (4 alike) : $bdroot/Digital variable notch fitlers  Ts=Ts  zeta=zeta
  Divide : Product  Inputs=*/
  Gain1 : Gain  Gain=4*pi*fn
  Gain2 : Gain  Gain=4*Ts*fn
  Multiply{1,4..5,8..16} (12 alike) : Product
  Mux{1..4} (4 alike) : Mux  Inputs=[2 1]
  Rate Transition1 : RateTransition  OutPortSampleTime=Ts
  Rate Transition2 : RateTransition  OutPortSampleTime=Ts
  Rate Transition3 : RateTransition  InitialCondition=1  OutPortSampleTime=Ts
  Rate Transition4 : RateTransition  OutPortSampleTime=Ts
  Saturation : Saturate  UpperLimit=inf  LowerLimit=0.000001
  Selector{1..3,5,9..16} (12 alike) : Selector  InputPortWidth=3  IndexOptions=Index vector (dialog)  Indices=[1 2]  OutputSizes=1
  Selector4 : Selector  InputPortWidth=3  IndexOptions=Index vector (dialog)  Indices=[1 3 2]  OutputSizes=1
  Selector7 : Selector  InputPortWidth=3  IndexOptions=Index vector (dialog)  Indices=[1 3 2]  OutputSizes=1
  Sum{2,4..6} (4 alike) : Sum  Inputs=+++
  Terminator : Terminator
  Terminator1 : Terminator
  Terminator2 : Terminator
  abc to Alpha-Beta-Zero{,1..3} (4 alike) : powerlib_meascontrol/Transformations/abc to Alpha-Beta-Zero
      settings: SourceProductName=Simscape Power Systems
  abc to dq{0..1,4..5} (4 alike) : powerlib_meascontrol/Transformations/abc to dq0  Alignment=90 degrees behind phase A axis
  alphabeta_DSC{,1..3} (4 alike) : $bdroot/alphabeta_DSC  Ts=Ts  nmax=round(1/(4*fmin*Ts))
  dq_DSC{,1,4..5} (4 alike) : $bdroot/dq_DSC  Ts=Ts  nmax=round(1/(4*fmin*Ts))
  vdq : Outport
  idq : Outport  Port=2
  vdq_pos : Outport  Port=3
  idq_pos : Outport  Port=4
  vdq_neg : Outport  Port=5
  idq_neg : Outport  Port=6
  wires:
  wt/1 -> Rate Transition2/1
  Selector5/1 -> Digital variable notch fitlers4/1, vdq/1, dq_DSC/1  "dq"
  abc to dq0/1 -> Selector5/1
  vabc/1 -> Rate Transition1/1
  iabc/1 -> Rate Transition4/1
  Digital variable notch fitlers4/1 -> Multiply5/2  "notch"
  Sum2/1 -> vdq_pos/1  "dq_pos"
  Rate Transition2/1 -> [wt]
  [wt] -> abc to dq0/2
  Divide/1 -> [N]  "N"
  Rate Transition1/1 -> Selector7/1, [vabc]
  Selector7/1 -> [vacb]
  Rate Transition4/1 -> Selector4/1, [iabc]
  Selector4/1 -> [iacb]
  Gain2/1 -> Saturation/1
  Saturation/1 -> Divide/2
  Constant/1 -> Divide/1
  Rate Transition3/1 -> Gain1/1, Gain2/1
  w_pu/1 -> Rate Transition3/1
  Gain1/1 -> [wnotch]
  [wnotch] -> Digital variable notch fitlers4/2
  [Notch] -> Multiply5/1
  Multiply4/1 -> Sum2/2
  [DSCdq] -> Multiply4/1
  Multiply5/1 -> Sum2/1
  [N] -> dq_DSC/2
  dq_DSC/1 -> Multiply4/2  "DSCdq"
  3waySelector/1 -> [Notch]
  3waySelector/2 -> Terminator/1
  3waySelector/4 -> Terminator1/1
  3waySelector/6 -> Terminator2/1
  Constant1/1 -> Mux1/2
  Alpha-Beta-Zero to dq0/1 -> Selector11/1
  [N] -> alphabeta_DSC/2
  [vabc] -> abc to Alpha-Beta-Zero/1, abc to dq0/1
  [wt] -> Alpha-Beta-Zero to dq0/2
  Mux1/1 -> Alpha-Beta-Zero to dq0/1
  abc to Alpha-Beta-Zero/1 -> Selector2/1
  Selector2/1 -> alphabeta_DSC/1  "alphabeta"
  alphabeta_DSC/1 -> Mux1/1
  3waySelector/5 -> [DSCdq]
  0:Notch,1:DSC,2:DSCdq/1 -> 3waySelector/1
  Selector11/1 -> Multiply8/2  "DSCab"
  [DSCab] -> Multiply8/1
  3waySelector/3 -> [DSCab]
  Multiply8/1 -> Sum2/3
  Selector1/1 -> Multiply10/2
  [DSCab] -> Multiply10/1
  abc to Alpha-Beta-Zero2/1 -> Selector9/1
  Selector9/1 -> alphabeta_DSC2/1  "alphabeta"
  Mux3/1 -> Alpha-Beta-Zero to dq2/1
  [N] -> alphabeta_DSC2/2
  Alpha-Beta-Zero to dq2/1 -> Selector1/1
  [wt] -> Alpha-Beta-Zero to dq2/2
  alphabeta_DSC2/1 -> Mux3/1
  Constant3/1 -> Mux3/2
  [Notch] -> Multiply9/1
  [N] -> dq_DSC1/2
  dq_DSC1/1 -> Multiply1/2
  Multiply1/1 -> Sum4/2
  Multiply9/1 -> Sum4/1
  Sum4/1 -> idq_pos/1  "dq_pos"
  [DSCdq] -> Multiply1/1
  [wnotch] -> Digital variable notch fitlers1/2
  [wt] -> abc to dq1/2
  [iabc] -> abc to Alpha-Beta-Zero2/1, abc to dq1/1
  Digital variable notch fitlers1/1 -> Multiply9/2  "dq"
  Selector10/1 -> idq/1, Digital variable notch fitlers1/1, dq_DSC1/1  "dq"
  Multiply10/1 -> Sum4/3
  abc to dq1/1 -> Selector10/1
  Selector13/1 -> Multiply15/2
  abc to Alpha-Beta-Zero1/1 -> Selector14/1
  [N] -> alphabeta_DSC1/2
  Alpha-Beta-Zero to dq1/1 -> Selector13/1
  [wt] -> Alpha-Beta-Zero to dq1/2
  alphabeta_DSC1/1 -> Mux2/1
  Constant2/1 -> Mux2/2
  [Notch] -> Multiply14/1
  [N] -> dq_DSC4/2
  Multiply14/1 -> Sum5/1
  Sum5/1 -> vdq_neg/1  "dq_pos"
  [DSCdq] -> Multiply13/1
  [wt] -> abc to dq4/2
  [vacb] -> abc to Alpha-Beta-Zero1/1, abc to dq4/1
  Selector3/1 -> Multiply12/2
  abc to dq5/1 -> Selector12/1
  Mux2/1 -> Alpha-Beta-Zero to dq1/1
  Multiply12/1 -> Sum6/3
  [wt] -> abc to dq5/2
  [DSCdq] -> Multiply11/1
  Digital variable notch fitlers6/1 -> Multiply14/2  "dq"
  [wnotch] -> Digital variable notch fitlers3/2
  [N] -> dq_DSC5/2
  dq_DSC5/1 -> Multiply11/2
  Multiply11/1 -> Sum6/2
  [Notch] -> Multiply16/1
  Multiply16/1 -> Sum6/1
  [N] -> alphabeta_DSC3/2
  Digital variable notch fitlers3/1 -> Multiply16/2  "dq"
  Multiply13/1 -> Sum5/2
  Constant4/1 -> Mux4/2
  Selector15/1 -> Digital variable notch fitlers6/1, dq_DSC4/1  "dq"
  [wt] -> Alpha-Beta-Zero to dq3/2
  Selector12/1 -> Digital variable notch fitlers3/1, dq_DSC5/1  "dq"
  abc to dq4/1 -> Selector15/1
  Alpha-Beta-Zero to dq3/1 -> Selector3/1
  [DSCab] -> Multiply15/1
  abc to Alpha-Beta-Zero3/1 -> Selector16/1
  Mux4/1 -> Alpha-Beta-Zero to dq3/1
  Selector14/1 -> alphabeta_DSC1/1  "alphabeta"
  alphabeta_DSC3/1 -> Mux4/1
  dq_DSC4/1 -> Multiply13/2
  [DSCab] -> Multiply12/1
  Sum6/1 -> idq_neg/1  "dq_pos"
  [iacb] -> abc to Alpha-Beta-Zero3/1, abc to dq5/1
  Multiply15/1 -> Sum5/3
  Selector16/1 -> alphabeta_DSC3/1  "alphabeta"
  [wnotch] -> Digital variable notch fitlers6/2

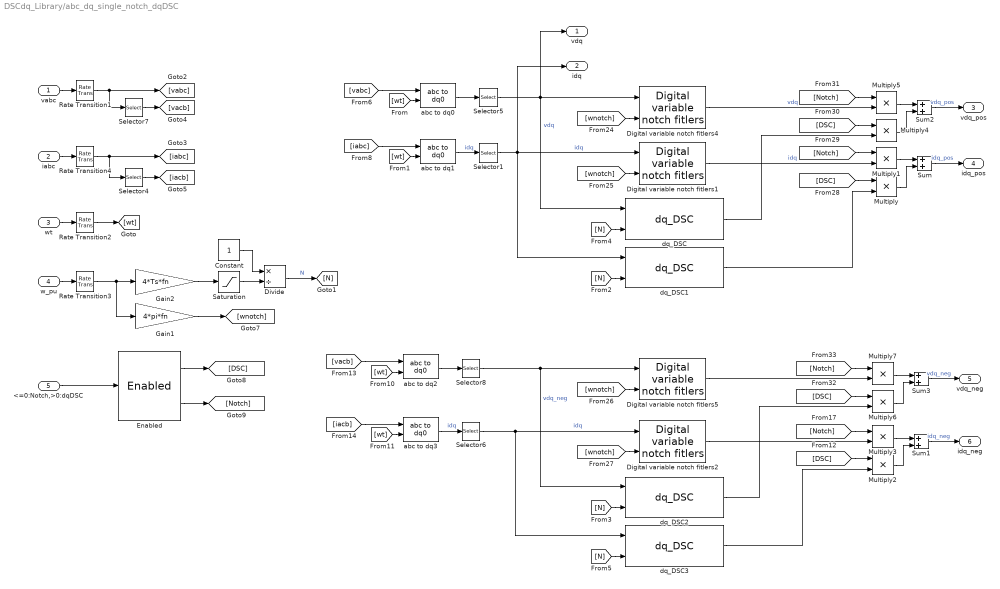
== system DSCdq_Library/abc_dq_single_notch_dqDSC ==
  vabc : Inport
  iabc : Inport  Port=2
  wt : Inport  Port=3
  w_pu : Inport  Port=4
  <=0:Notch,>0:dqDSC : Inport  Port=5
  Constant : Constant
  Digital variable notch fitlers{1..2,4..5} (4 alike) : $bdroot/Digital variable notch fitlers  Ts=Ts  zeta=zeta
  Divide : Product  Inputs=*/
  Enabled : $bdroot/Enabled
  Gain1 : Gain  Gain=4*pi*fn
  Gain2 : Gain  Gain=4*Ts*fn
  Multiply{,1..7} (8 alike) : Product
  Rate Transition1 : RateTransition  OutPortSampleTime=Ts
  Rate Transition2 : RateTransition  OutPortSampleTime=Ts
  Rate Transition3 : RateTransition  InitialCondition=1  OutPortSampleTime=Ts
  Rate Transition4 : RateTransition  OutPortSampleTime=Ts
  Saturation : Saturate  UpperLimit=inf  LowerLimit=0.000001
  Selector{1,5..6,8} (4 alike) : Selector  InputPortWidth=3  IndexOptions=Index vector (dialog)  Indices=[1 2]  OutputSizes=1
  Selector4 : Selector  InputPortWidth=3  IndexOptions=Index vector (dialog)  Indices=[1 3 2]  OutputSizes=1
  Selector7 : Selector  InputPortWidth=3  IndexOptions=Index vector (dialog)  Indices=[1 3 2]  OutputSizes=1
  Sum{,1..3} (4 alike) : Sum
  abc to dq{0..3} (4 alike) : powerlib_meascontrol/Transformations/abc to dq0  Alignment=90 degrees behind phase A axis
  dq_DSC{,1..3} (4 alike) : $bdroot/dq_DSC  Ts=Ts  nmax=round(1/(4*fmin*Ts))
  vdq : Outport
  idq : Outport  Port=2
  vdq_pos : Outport  Port=3
  idq_pos : Outport  Port=4
  vdq_neg : Outport  Port=5
  idq_neg : Outport  Port=6
  wires:
  wt/1 -> Rate Transition2/1
  abc to dq1/1 -> Selector1/1  "idq"
  Selector5/1 -> Digital variable notch fitlers4/1, vdq/1, dq_DSC/1  "vdq"
  abc to dq0/1 -> Selector5/1
  Selector1/1 -> Digital variable notch fitlers1/1, idq/1, dq_DSC1/1  "idq"
  [vabc] -> abc to dq0/1
  [iabc] -> abc to dq1/1
  vabc/1 -> Rate Transition1/1
  iabc/1 -> Rate Transition4/1
  Digital variable notch fitlers4/1 -> Multiply5/2  "vdq"
  Digital variable notch fitlers1/1 -> Multiply1/2  "idq"
  Sum2/1 -> vdq_pos/1  "vdq_pos"
  Sum/1 -> idq_pos/1  "idq_pos"
  Rate Transition2/1 -> [wt]
  [wt] -> abc to dq0/2
  [wt] -> abc to dq1/2
  Divide/1 -> [N]  "N"
  Rate Transition1/1 -> Selector7/1, [vabc]
  Selector7/1 -> [vacb]
  Rate Transition4/1 -> Selector4/1, [iabc]
  Selector4/1 -> [iacb]
  [wt] -> abc to dq3/2
  abc to dq2/1 -> Selector8/1
  Selector8/1 -> Digital variable notch fitlers5/1, dq_DSC2/1  "vdq_neg"
  [vacb] -> abc to dq2/1
  [wt] -> abc to dq2/2
  abc to dq3/1 -> Selector6/1  "idq"
  [iacb] -> abc to dq3/1
  Sum3/1 -> vdq_neg/1  "vdq_neg"
  Sum1/1 -> idq_neg/1  "idq_neg"
  Digital variable notch fitlers5/1 -> Multiply7/2
  Selector6/1 -> Digital variable notch fitlers2/1, dq_DSC3/1  "idq"
  Digital variable notch fitlers2/1 -> Multiply3/2
  dq_DSC3/1 -> Multiply2/2
  Gain2/1 -> Saturation/1
  Saturation/1 -> Divide/2
  Constant/1 -> Divide/1
  Rate Transition3/1 -> Gain1/1, Gain2/1
  w_pu/1 -> Rate Transition3/1
  Gain1/1 -> [wnotch]
  [wnotch] -> Digital variable notch fitlers4/2
  [wnotch] -> Digital variable notch fitlers1/2
  [wnotch] -> Digital variable notch fitlers5/2
  [wnotch] -> Digital variable notch fitlers2/2
  <=0:Notch,>0:dqDSC/1 -> Enabled/1
  Enabled/1 -> [DSC]
  Enabled/2 -> [Notch]
  [DSC] -> Multiply/1
  [Notch] -> Multiply1/1
  Multiply1/1 -> Sum/1
  Multiply/1 -> Sum/2
  [Notch] -> Multiply3/1
  [DSC] -> Multiply2/1
  Multiply3/1 -> Sum1/1
  Multiply2/1 -> Sum1/2
  [Notch] -> Multiply5/1
  Multiply4/1 -> Sum2/2
  [DSC] -> Multiply4/1
  Multiply5/1 -> Sum2/1
  [Notch] -> Multiply7/1
  Multiply6/1 -> Sum3/2
  [DSC] -> Multiply6/1
  Multiply7/1 -> Sum3/1
  [N] -> dq_DSC/2
  [N] -> dq_DSC1/2
  dq_DSC1/1 -> Multiply/2
  [N] -> dq_DSC3/2
  dq_DSC/1 -> Multiply4/2
  [N] -> dq_DSC2/2
  dq_DSC2/1 -> Multiply6/2

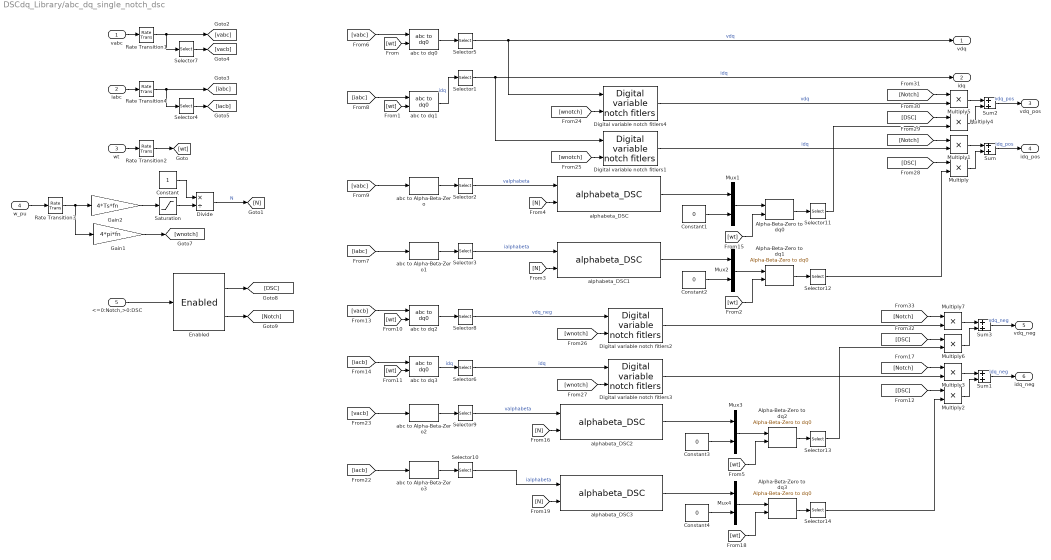
== system DSCdq_Library/abc_dq_single_notch_dsc ==
  vabc : Inport
  iabc : Inport  Port=2
  wt : Inport  Port=3
  w_pu : Inport  Port=4
  <=0:Notch,>0:DSC : Inport  Port=5
  Alpha-Beta-Zero to dq{0..3} (4 alike) : powerlib_meascontrol/Transformations/Alpha-Beta-Zero to dq0  Alignment=90 degrees behind phase A axis
      settings: SourceProductName=Simscape Power Systems
  Constant : Constant
  Constant{1..4} (4 alike) : Constant  Value=0
  Digital variable notch fitlers{1..4} (4 alike) : $bdroot/Digital variable notch fitlers  Ts=Ts  zeta=zeta
  Divide : Product  Inputs=*/
  Enabled : $bdroot/Enabled
  Gain1 : Gain  Gain=4*pi*fn
  Gain2 : Gain  Gain=4*Ts*fn
  Multiply{,1..7} (8 alike) : Product
  Mux{1..4} (4 alike) : Mux  Inputs=[2 1]
  Rate Transition1 : RateTransition  OutPortSampleTime=Ts
  Rate Transition2 : RateTransition  OutPortSampleTime=Ts
  Rate Transition3 : RateTransition  InitialCondition=1  OutPortSampleTime=Ts
  Rate Transition4 : RateTransition  OutPortSampleTime=Ts
  Saturation : Saturate  UpperLimit=inf  LowerLimit=0.000001
  Selector{1..3,5..6,8..14} (12 alike) : Selector  InputPortWidth=3  IndexOptions=Index vector (dialog)  Indices=[1 2]  OutputSizes=1
  Selector4 : Selector  InputPortWidth=3  IndexOptions=Index vector (dialog)  Indices=[1 3 2]  OutputSizes=1
  Selector7 : Selector  InputPortWidth=3  IndexOptions=Index vector (dialog)  Indices=[1 3 2]  OutputSizes=1
  Sum{,1..3} (4 alike) : Sum
  abc to Alpha-Beta-Zero{,1..3} (4 alike) : powerlib_meascontrol/Transformations/abc to Alpha-Beta-Zero
      settings: SourceProductName=Simscape Power Systems
  abc to dq{0..3} (4 alike) : powerlib_meascontrol/Transformations/abc to dq0  Alignment=90 degrees behind phase A axis
  alphabeta_DSC{,1..3} (4 alike) : $bdroot/alphabeta_DSC  Ts=Ts  nmax=round(1/(4*fmin*Ts))
  vdq : Outport
  idq : Outport  Port=2
  vdq_pos : Outport  Port=3
  idq_pos : Outport  Port=4
  vdq_neg : Outport  Port=5
  idq_neg : Outport  Port=6
  wires:
  wt/1 -> Rate Transition2/1
  abc to dq1/1 -> Selector1/1  "idq"
  Selector5/1 -> Digital variable notch fitlers4/1, vdq/1  "vdq"
  abc to dq0/1 -> Selector5/1
  Selector1/1 -> Digital variable notch fitlers1/1, idq/1  "idq"
  abc to Alpha-Beta-Zero/1 -> Selector2/1
  abc to Alpha-Beta-Zero1/1 -> Selector3/1
  Selector11/1 -> Multiply4/2
  Selector3/1 -> alphabeta_DSC1/1  "ialphabeta"
  [vabc] -> abc to dq0/1
  [iabc] -> abc to dq1/1
  vabc/1 -> Rate Transition1/1
  iabc/1 -> Rate Transition4/1
  Selector2/1 -> alphabeta_DSC/1  "valphabeta"
  Digital variable notch fitlers4/1 -> Multiply5/2  "vdq"
  Digital variable notch fitlers1/1 -> Multiply1/2  "idq"
  Selector12/1 -> Multiply/2
  Sum2/1 -> vdq_pos/1  "vdq_pos"
  Sum/1 -> idq_pos/1  "idq_pos"
  Rate Transition2/1 -> [wt]
  [wt] -> abc to dq0/2
  [wt] -> abc to dq1/2
  Divide/1 -> [N]  "N"
  Rate Transition1/1 -> Selector7/1, [vabc]
  Selector7/1 -> [vacb]
  Rate Transition4/1 -> Selector4/1, [iabc]
  Selector4/1 -> [iacb]
  [vabc] -> abc to Alpha-Beta-Zero/1
  [iabc] -> abc to Alpha-Beta-Zero1/1
  [wt] -> abc to dq3/2
  abc to dq2/1 -> Selector8/1
  Selector8/1 -> Digital variable notch fitlers2/1  "vdq_neg"
  [vacb] -> abc to dq2/1
  [wt] -> abc to dq2/2
  abc to dq3/1 -> Selector6/1  "idq"
  [iacb] -> abc to dq3/1
  Sum3/1 -> vdq_neg/1  "vdq_neg"
  Sum1/1 -> idq_neg/1  "idq_neg"
  Digital variable notch fitlers2/1 -> Multiply7/2
  Selector6/1 -> Digital variable notch fitlers3/1  "idq"
  Digital variable notch fitlers3/1 -> Multiply3/2
  abc to Alpha-Beta-Zero3/1 -> Selector10/1
  Selector10/1 -> alphabeta_DSC3/1  "ialphabeta"
  abc to Alpha-Beta-Zero2/1 -> Selector9/1
  [iacb] -> abc to Alpha-Beta-Zero3/1
  [vacb] -> abc to Alpha-Beta-Zero2/1
  Alpha-Beta-Zero to dq2/1 -> Selector13/1
  Selector9/1 -> alphabeta_DSC2/1  "valphabeta"
  Alpha-Beta-Zero to dq3/1 -> Selector14/1
  Gain2/1 -> Saturation/1
  Saturation/1 -> Divide/2
  Constant/1 -> Divide/1
  Rate Transition3/1 -> Gain1/1, Gain2/1
  w_pu/1 -> Rate Transition3/1
  Gain1/1 -> [wnotch]
  [wnotch] -> Digital variable notch fitlers4/2
  [wnotch] -> Digital variable notch fitlers1/2
  [wnotch] -> Digital variable notch fitlers2/2
  [wnotch] -> Digital variable notch fitlers3/2
  <=0:Notch,>0:DSC/1 -> Enabled/1
  Enabled/1 -> [DSC]
  Enabled/2 -> [Notch]
  [DSC] -> Multiply/1
  [Notch] -> Multiply1/1
  Multiply1/1 -> Sum/1
  Multiply/1 -> Sum/2
  [Notch] -> Multiply3/1
  [DSC] -> Multiply2/1
  Multiply3/1 -> Sum1/1
  Multiply2/1 -> Sum1/2
  [Notch] -> Multiply5/1
  Multiply4/1 -> Sum2/2
  [DSC] -> Multiply4/1
  Multiply5/1 -> Sum2/1
  [Notch] -> Multiply7/1
  Multiply6/1 -> Sum3/2
  [DSC] -> Multiply6/1
  Multiply7/1 -> Sum3/1
  Mux1/1 -> Alpha-Beta-Zero to dq0/1
  Alpha-Beta-Zero to dq0/1 -> Selector11/1
  [wt] -> Alpha-Beta-Zero to dq0/2
  Constant1/1 -> Mux1/2
  alphabeta_DSC/1 -> Mux1/1
  [N] -> alphabeta_DSC/2
  [wt] -> Alpha-Beta-Zero to dq1/2
  Alpha-Beta-Zero to dq1/1 -> Selector12/1
  Mux2/1 -> Alpha-Beta-Zero to dq1/1
  alphabeta_DSC1/1 -> Mux2/1
  Constant2/1 -> Mux2/2
  [N] -> alphabeta_DSC1/2
  Mux3/1 -> Alpha-Beta-Zero to dq2/1
  Constant3/1 -> Mux3/2
  [wt] -> Alpha-Beta-Zero to dq2/2
  [N] -> alphabeta_DSC2/2
  alphabeta_DSC2/1 -> Mux3/1
  Mux4/1 -> Alpha-Beta-Zero to dq3/1
  Constant4/1 -> Mux4/2
  [wt] -> Alpha-Beta-Zero to dq3/2
  [N] -> alphabeta_DSC3/2
  alphabeta_DSC3/1 -> Mux4/1
  Selector13/1 -> Multiply6/2
  Selector14/1 -> Multiply2/2

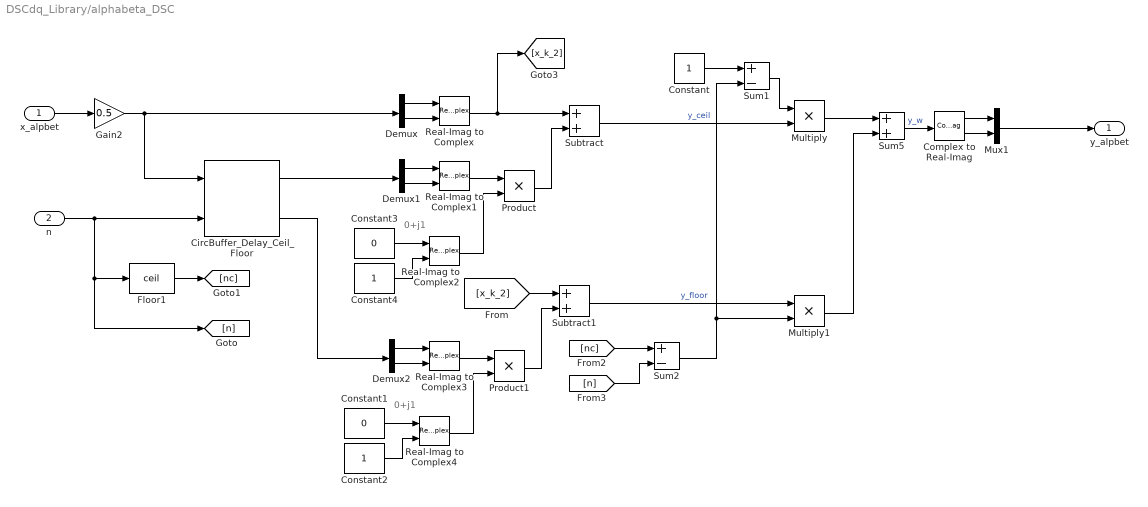
== system DSCdq_Library/alphabeta_DSC ==
  note: 0+j1
  note: 0+j1
  x_alpbet : Inport
  n : Inport  Port=2
  CircBuffer_Delay_Ceil_Floor : $bdroot/CircBuffer_Delay_Ceil_Floor  Ts=Ts  nmax=200
  Complex to Real-Imag : ComplexToRealImag
  Constant : Constant
  Constant1 : Constant  Value=0
  Constant2 : Constant
  Constant3 : Constant  Value=0
  Constant4 : Constant
  Demux : Demux  Outputs=2
  Demux1 : Demux  Outputs=2
  Demux2 : Demux  Outputs=2
  Floor1 : Rounding  Operator=ceil
  Gain2 : Gain  Gain=0.5
  Multiply : Product
  Multiply1 : Product
  Mux1 : Mux  Inputs=[1 1]
  Product : Product
  Product1 : Product
  Real-Imag to Complex{,1..4} (5 alike) : RealImagToComplex
  Subtract : Sum
  Subtract1 : Sum
  Sum1 : Sum  Inputs=+-
  Sum2 : Sum  Inputs=+-
  Sum5 : Sum
  y_alpbet : Outport
  wires:
  Complex to Real-Imag/2 -> Mux1/2
  Mux1/1 -> y_alpbet/1
  Demux/1 -> Real-Imag to Complex/1
  Product/1 -> Subtract/2
  x_alpbet/1 -> Gain2/1
  Demux/2 -> Real-Imag to Complex/2
  CircBuffer_Delay_Ceil_Floor/1 -> Demux1/1
  Complex to Real-Imag/1 -> Mux1/1
  Demux1/2 -> Real-Imag to Complex1/2
  Constant4/1 -> Real-Imag to Complex2/2
  n/1 -> Floor1/1, [n], CircBuffer_Delay_Ceil_Floor/2
  Real-Imag to Complex/1 -> [x_k_2], Subtract/1
  Constant3/1 -> Real-Imag to Complex2/1
  Real-Imag to Complex1/1 -> Product/1
  Demux1/1 -> Real-Imag to Complex1/1
  Real-Imag to Complex2/1 -> Product/2
  [nc] -> Sum2/1
  Sum2/1 -> Multiply1/2, Sum1/2
  Subtract1/1 -> Multiply1/1  "y_floor"
  Subtract/1 -> Multiply/2  "y_ceil"
  Multiply/1 -> Sum5/1
  Multiply1/1 -> Sum5/2
  Sum1/1 -> Multiply/1
  [n] -> Sum2/2
  Constant/1 -> Sum1/1
  Floor1/1 -> [nc]
  Demux2/1 -> Real-Imag to Complex3/1
  Constant1/1 -> Real-Imag to Complex4/1
  Demux2/2 -> Real-Imag to Complex3/2
  Constant2/1 -> Real-Imag to Complex4/2
  Product1/1 -> Subtract1/2
  Real-Imag to Complex3/1 -> Product1/1
  Real-Imag to Complex4/1 -> Product1/2
  CircBuffer_Delay_Ceil_Floor/2 -> Demux2/1
  Gain2/1 -> Demux/1, CircBuffer_Delay_Ceil_Floor/1
  [x_k_2] -> Subtract1/1
  Sum5/1 -> Complex to Real-Imag/1  "y_w"
